simulink model "plant_tests_dz_no_reset"  (R2015a)
settings: Solver=ode3  StartTime=0.0  StopTime=T  RelTol=1e-3
values from neighbouring files (symbols this model uses):
  A = stateModelMatrices(1:l-1, 1:l-1)    [controller_design_1.m]    (also in controller_design_2.m)
  B = stateModelMatrices(1:l-1, l)    [controller_design_1.m]    (also in controller_design_2.m)
  C = stateModelMatrices(l, 1:l-1)    [controller_design_1.m]    (also in controller_design_2.m)
  Ke = -3.30696316959    [sensor_param.mat]
  Kp = 34.1808066759    [sensor_param.mat]
  Nbar = Nu+K*Nx    [controller_design_1.m]    (also in controller_design_2.m)
  Ts = 0.02    [controller_design_1.m]    (also in controller_design_2.m)
undefined symbols (not defined in the file or in its folder): K, M, MIO, National_Instruments, PCI
libraries: sldrtlib x2
settings Model: SimulationMode=external  ExtModeTrigDuration=1000000  Creator=alunos  LastModifiedBy=alunos
settings DataIOCC: LimitDataPoints=off
settings HardwareCC: ProdIntDivRoundTo=Zero  ProdEndianess=LittleEndian  ProdHWDeviceType=Intel->x86/Pentium  TargetIntDivRoundTo=Zero  TargetEndianess=LittleEndian  TargetHWDeviceType=Intel->x86/Pentium
settings RTWCC: SystemTargetFile=rtwin.tlc  TemplateMakefile=rtwin.tmf  Description=Simulink Desktop Real-Time  RTWCompilerOptimization=on
settings CodeAppCC: MaxIdLength=95
settings RTWinTargetCC: TargetPreCompLibLocation=C:\Program Files\MATLAB\R2015a\toolbox\sldrt\lib\win32

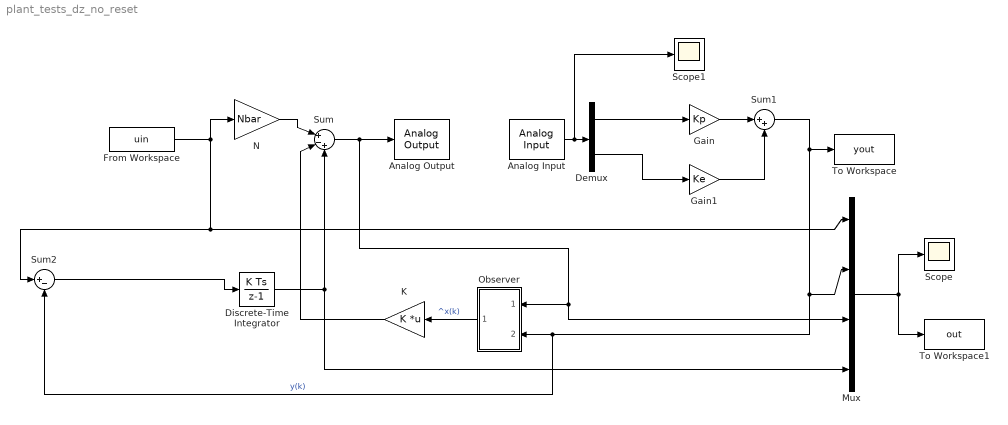
== system plant_tests_dz_no_reset ==
  Analog Input : sldrtlib/Analog Input  SampleTime=Ts  MaxMissedTicks=10  ShowMissedTicks=off  YieldWhenWaiting=off  DrvName=National_Instruments/PCI-MIO-16E-4  DrvAddress=4294967295  DrvOptions=[0 0 0 0 0 0]  Channels=[1 2]  RangeMode=1  VoltRange=1  DataType=1
      settings: AttributesFormatString=National Instruments\nPCI-MIO-16E-4 [auto]
  Analog Output : sldrtlib/Analog Output  SampleTime=Ts  MaxMissedTicks=10  ShowMissedTicks=off  YieldWhenWaiting=off  DrvName=National_Instruments/PCI-MIO-16E-4  DrvAddress=4294967295  DrvOptions=[0 0 0 0 0 0]  Channels=1  RangeMode=1  VoltRange=1  InitialValue=0  FinalValue=0
      settings: AttributesFormatString=National Instruments\nPCI-MIO-16E-4 [auto]
  Demux : Demux  Outputs=2
  Discrete-Time Integrator : DiscreteIntegrator  gainval=0.1  InitialConditionSetting=State (most efficient)  SampleTime=0.02
  From Workspace : FromWorkspace  VariableName=uin  SampleTime=Ts  OutputAfterFinalValue=Setting to zero
  Gain : Gain  Gain=Kp
  Gain1 : Gain  Gain=Ke
  K : Gain  Gain=K  Multiplication=Matrix(K*u)
  Mux : Mux
  N : Gain  Gain=Nbar
  Observer : Subsystem
  Scope : Scope
      settings: TimeRange=20  YMin=-40  YMax=45
  Scope1 : Scope
      settings: YMin=-1.32807  YMax=1.32791
  Sum : Sum  Inputs=|+-+
  Sum1 : Sum  Inputs=|++
  Sum2 : Sum  Inputs=|+-
  To Workspace : ToWorkspace  VariableName=yout  SampleTime=-1
  To Workspace1 : ToWorkspace  VariableName=out  SaveFormat=Structure With Time  SampleTime=-1
  wires:
  From Workspace/1 -> Mux/1, Sum2/1, N/1
  N/1 -> Sum/1
  Sum/1 -> Mux/3, Observer/1(In1), Analog Output/1
  K/1 -> Sum/2
  Observer/1(Out1) -> K/1  "^x(k)"
  Analog Input/1 -> Scope1/1, Demux/1
  Sum1/1 -> Sum2/2, Observer/2(In2), Mux/2, To Workspace/1  "y(k)"
  Demux/1 -> Gain/1
  Demux/2 -> Gain1/1
  Gain/1 -> Sum1/1
  Gain1/1 -> Sum1/2
  Mux/1 -> To Workspace1/1, Scope/1
  Discrete-Time Integrator/1 -> Mux/4, Sum/3
  Sum2/1 -> Discrete-Time Integrator/1

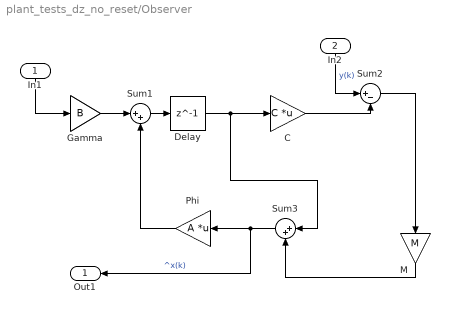
== system plant_tests_dz_no_reset/Observer ==
  In1 : Inport
  In2 : Inport  Port=2
  C : Gain  Gain=C  Multiplication=Matrix(K*u)
  Delay : Delay  DelayLength=1  InitialCondition=0  SampleTime=Ts
  Gamma : Gain  Gain=B
  M : Gain  Gain=M
  Phi : Gain  Gain=A  Multiplication=Matrix(K*u)
  Sum1 : Sum  Inputs=|++
  Sum2 : Sum  Inputs=|+-
  Sum3 : Sum  Inputs=|++
  Out1 : Outport
  wires:
  In1/1 -> Gamma/1
  In2/1 -> Sum2/1  "y(k)"
  Gamma/1 -> Sum1/1
  Sum1/1 -> Delay/1
  Delay/1 -> Sum3/1, C/1
  Sum2/1 -> M/1
  C/1 -> Sum2/2
  Phi/1 -> Sum1/2
  Sum3/1 -> Out1/1, Phi/1  "^x(k)"
  M/1 -> Sum3/2
